simulink library "PB_Library_Master"  (R2020b)
settings: Solver=VariableStepAuto  StartTime=0.0  StopTime=10.0  RelTol=1e-3
undefined symbols (not defined in the file): A_M, B_M, E0_M, f_sw, K_M, Q_M, Q_rr, r_c, r_D, R_M, SOC_Init_M, u_ce0, u_D0
libraries: $bdroot x7, Lib_PF_BusLoadDC_TMATS x3, Lib_Dyn_StateSpace_EMTAT x3, TemperatureBlock x1
(part 2 of 3)

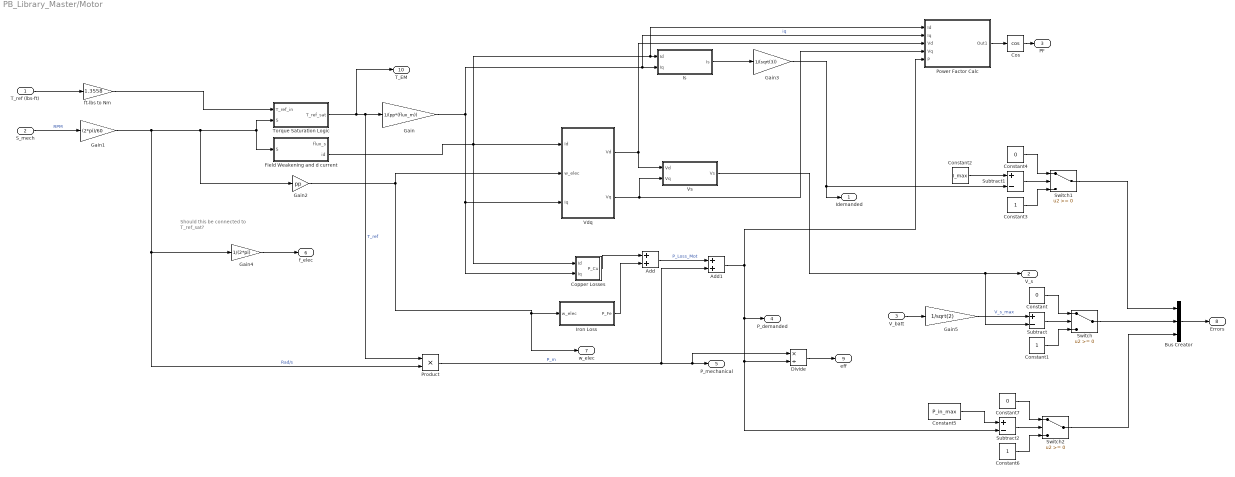
== system PB_Library_Master/Motor ==
  note: Should this be connected
      | to T_ref_sat?
  T_ref (lbs-ft) : Inport
  S_mech : Inport  Port=2
  V_batt : Inport  Port=3
  Add : Sum
  Add1 : Sum
  Bus Creator : BusCreator  Inputs=3
  Constant : Constant  Value=0
  Constant1 : Constant
  Constant2 : Constant  Value=I_max
  Constant3 : Constant
  Constant4 : Constant  Value=0
  Constant5 : Constant  Value=P_in_max
  Constant6 : Constant
  Constant7 : Constant  Value=0
  Copper Losses : Subsystem
  Cos : Trigonometry  Operator=cos
  Divide : Product  Inputs=*/
  "Field Weakening and d current " : Subsystem
  Gain : Gain  Gain=1/(pp*(flux_m))
  Gain1 : Gain  Gain=(2*pi)/60
  Gain2 : Gain  Gain=pp
  Gain3 : Gain  Gain=1/(sqrt(3))
  Gain4 : Gain  Gain=1/(2*pi)
  Gain5 : Gain  Gain=1/sqrt(2)
  Iron Loss : Subsystem
  Is : Subsystem
  "Power Factor Calc " : Subsystem
  Product : Product
  Subtract : Sum  Inputs=+-
  Subtract1 : Sum  Inputs=+-
  Subtract2 : Sum  Inputs=+-
  Switch : Switch
  Switch1 : Switch
  Switch2 : Switch
  Torque Saturation Logic : Subsystem
  Vdq : Subsystem
  Vs : Subsystem
  ft-lbs to Nm : Gain  Gain=1.3558
  Idemanded : Outport  VectorParamsAs1DForOutWhenUnconnected=off
  V_s : Outport  Port=2  VectorParamsAs1DForOutWhenUnconnected=off
  PF : Outport  Port=3  VectorParamsAs1DForOutWhenUnconnected=off
  P_demanded : Outport  Port=4  VectorParamsAs1DForOutWhenUnconnected=off
  P_mechanical : Outport  Port=5  VectorParamsAs1DForOutWhenUnconnected=off
  f_elec : Outport  Port=6  VectorParamsAs1DForOutWhenUnconnected=off
  w_elec : Outport  Port=7  VectorParamsAs1DForOutWhenUnconnected=off
  Errors : Outport  Port=8  VectorParamsAs1DForOutWhenUnconnected=off
  eff : Outport  Port=9  VectorParamsAs1DForOutWhenUnconnected=off
  T_EM : Outport  Port=10  VectorParamsAs1DForOutWhenUnconnected=off
  wires:
  S_mech/1 -> Gain1/1  "RPM"
  T_ref (lbs-ft)/1 -> ft-lbs to Nm/1
  "Field Weakening and d current "/2(id) -> Copper Losses/1(Id), "Power Factor Calc "/1(Id), Is/1(Id), Vdq/1(Id)
  Gain3/1 -> Subtract1/2, Idemanded/1
  Gain2/1 -> Vdq/2(w_elec), w_elec/1, Iron Loss/1(w_elec)
  Torque Saturation Logic/1(T_ref_sat) -> T_EM/1, Product/1, Gain/1  "T_ref"
  Gain/1 -> "Power Factor Calc "/2(Iq), Is/2(Iq), Copper Losses/2(Iq), Vdq/3(Iq)  "iq"
  Gain1/1 -> Gain4/1, Product/2, Gain2/1, "Field Weakening and d current "/1(S), Torque Saturation Logic/2(S)  "Rad/s"
  Copper Losses/1(P_Cu) -> Add/1
  Iron Loss/1(P_Fe) -> Add/2
  Add/1 -> Add1/1  "P_Loss_Mot"
  Product/1 -> Add1/2, Divide/1, P_mechanical/1  "P_m"
  Vdq/1(Vd) -> Vs/1(Vd), "Power Factor Calc "/3(Vd)
  Vdq/2(Vq) -> "Power Factor Calc "/4(Vq), Vs/2(Vq)
  Is/1(Is) -> Gain3/1
  Vs/1(Vs) -> Subtract/2, V_s/1
  "Power Factor Calc "/1(Out1) -> Cos/1
  Add1/1 -> Divide/2, Subtract2/2, P_demanded/1, "Power Factor Calc "/5(P)
  Gain4/1 -> f_elec/1
  V_batt/1 -> Gain5/1
  Gain5/1 -> Subtract/1  "V_s_max"
  Subtract/1 -> Switch/2
  Constant/1 -> Switch/1
  Constant1/1 -> Switch/3
  Switch/1 -> Bus Creator/2
  Constant2/1 -> Subtract1/1
  Switch1/1 -> Bus Creator/1
  Constant3/1 -> Switch1/3
  Constant4/1 -> Switch1/1
  Subtract1/1 -> Switch1/2
  Constant7/1 -> Switch2/1
  Constant5/1 -> Subtract2/1
  Subtract2/1 -> Switch2/2
  Constant6/1 -> Switch2/3
  Divide/1 -> eff/1
  Cos/1 -> PF/1
  Bus Creator/1 -> Errors/1
  Switch2/1 -> Bus Creator/3
  ft-lbs to Nm/1 -> Torque Saturation Logic/1(T_ref_in)

== system PB_Library_Master/Rankine to Celsius ==
  Rankine : Inport
  Add : Sum  Inputs=+-
  Constant : Constant  Value=491.67
  Constant1 : Constant  Value=1.8
  Divide : Product  Inputs=*/
  Celsius : Outport
  wires:
  Divide/1 -> Celsius/1
  Rankine/1 -> Add/1
  Constant/1 -> Add/2
  Add/1 -> Divide/1
  Constant1/1 -> Divide/2

== system PB_Library_Master/Resistor_I ==
  Iout : Inport
  Idemand : Inport  Port=2
  Temp (Rankine) : Inport  Port=3  Unit=degC
  Multiply : Product
  Multiply1 : Product
  Rankine to Celsius : $bdroot/Rankine to Celsius  SystemSampleTime=-1  VariantActivationTime=update diagram  Latency=0  AutoFrameSizeCalculation=off
  Terminator : Terminator
  VDrop : Outport  VectorParamsAs1DForOutWhenUnconnected=off
  Iin : Outport  Port=2  VectorParamsAs1DForOutWhenUnconnected=off
  Heat : Outport  Port=3  VectorParamsAs1DForOutWhenUnconnected=off
  wires:
  Iout/1 -> Multiply/2, Multiply1/2, Iin/1
  Multiply/1 -> VDrop/1, Multiply1/1
  Idemand/1 -> Multiply/1
  Multiply1/1 -> Heat/1
  Temp (Rankine)/1 -> Rankine to Celsius/1
  Rankine to Celsius/1 -> Terminator/1

== system PB_Library_Master/Resistor_V ==
  "VDrop " : Inport
  "Resistance " : Inport  Port=2
  Temp : Inport  Port=3  Unit=degC
  Divide : Product  Inputs=*/
  Multiply1 : Product
  Rankine to Celsius : $bdroot/Rankine to Celsius  SystemSampleTime=-1  VariantActivationTime=update diagram  Latency=0  AutoFrameSizeCalculation=off
  Terminator : Terminator
  Iin : Outport  VectorParamsAs1DForOutWhenUnconnected=off
  Heat : Outport  Port=2  VectorParamsAs1DForOutWhenUnconnected=off
  wires:
  Multiply1/1 -> Heat/1
  "VDrop "/1 -> Multiply1/1, Divide/1
  "Resistance "/1 -> Divide/2
  Divide/1 -> Multiply1/2, Iin/1
  Temp/1 -> Rankine to Celsius/1
  Rankine to Celsius/1 -> Terminator/1

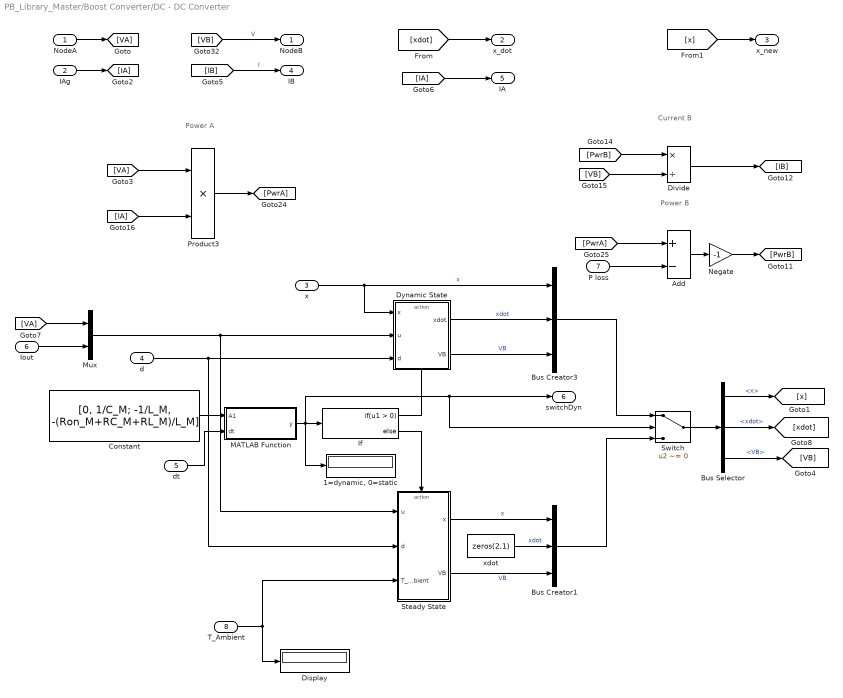
== system PB_Library_Master/Boost Converter/DC - DC Converter ==
  note: Power B
  note: Current B
  note: Power A
  NodeA : Inport
  IAg : Inport  Port=2
  x : Inport  Port=3
  d : Inport  Port=4
  dt : Inport  Port=5
  Iout : Inport  Port=6
  P loss : Inport  Port=7
  "T_Ambient " : Inport  Port=8
  " Dynamic State" : Subsystem  TreatAsAtomicUnit=on
  "1=dynamic, 0=static" : Display
  Add : Sum  Inputs=+-
  Bus Creator1 : BusCreator  Inputs=3
  Bus Creator3 : BusCreator  Inputs=3
  Bus Selector : BusSelector  OutputSignals=x,xdot,VB
  Constant : Constant  Value=[0, 1/C_M; -1/L_M, -(Ron_M+RC_M+RL_M)/L_M]  VectorParams1D=off
  Display : Display
  Divide : Product  Inputs=*/
  If : If
  MATLAB Function : MATLAB Function  TreatAsAtomicUnit=on
  Mux : Mux  Inputs=2
  Negate : Gain  Gain=-1
  Product3 : Product
  Steady State : Subsystem  TreatAsAtomicUnit=on
  Switch : Switch  Criteria=u2 ~= 0
  xdot : Constant  Value=zeros(2,1)  VectorParams1D=off
  NodeB : Outport  VectorParamsAs1DForOutWhenUnconnected=off
  x_dot : Outport  Port=2  VectorParamsAs1DForOutWhenUnconnected=off
  x_new : Outport  Port=3  VectorParamsAs1DForOutWhenUnconnected=off
  IB : Outport  Port=4  VectorParamsAs1DForOutWhenUnconnected=off
  IA : Outport  Port=5  VectorParamsAs1DForOutWhenUnconnected=off
  switchDyn : Outport  Port=6  VectorParamsAs1DForOutWhenUnconnected=off
  wires:
  "T_Ambient "/1 -> Steady State/3("T_Ambient "), Display/1
  Negate/1 -> [PwrB]
  Mux/1 -> " Dynamic State"/2(u), Steady State/1(u)
  Iout/1 -> Mux/2
  [VA] -> Mux/1
  [x] -> x_new/1
  Bus Creator3/1 -> Switch/1
  Bus Selector/1 -> [x]  "<x>"
  Bus Selector/2 -> [xdot]  "<xdot>"
  Bus Selector/3 -> [VB]  "<VB>"
  xdot/1 -> Bus Creator1/2  "xdot"
  Steady State/2(VB) -> Bus Creator1/3  "VB"
  " Dynamic State"/1(xdot) -> Bus Creator3/2  "xdot"
  " Dynamic State"/2(VB) -> Bus Creator3/3  "VB"
  Switch/1 -> Bus Selector/1
  Add/1 -> Negate/1
  P loss/1 -> Add/2
  [PwrA] -> Add/1
  [xdot] -> x_dot/1
  d/1 -> " Dynamic State"/3(d), Steady State/2(d)
  x/1 -> " Dynamic State"/1(x), Bus Creator3/1  "x"
  Steady State/1(x) -> Bus Creator1/1  "x"
  dt/1 -> MATLAB Function/2(dt)
  If/2 -> Steady State/Action
  Constant/1 -> MATLAB Function/1(A1)
  If/1 -> " Dynamic State"/Action
  MATLAB Function/1(y) -> If/1, switchDyn/1, Switch/2, "1=dynamic, 0=static"/1
  [IA] -> IA/1
  [IB] -> IB/1  "I"
  IAg/1 -> [IA]
  [VB] -> Divide/2
  Divide/1 -> [IB]
  [PwrB] -> Divide/1
  [IA] -> Product3/2
  NodeA/1 -> [VA]
  [VB] -> NodeB/1  "V"
  Product3/1 -> [PwrA]
  [VA] -> Product3/1
  Bus Creator1/1 -> Switch/3

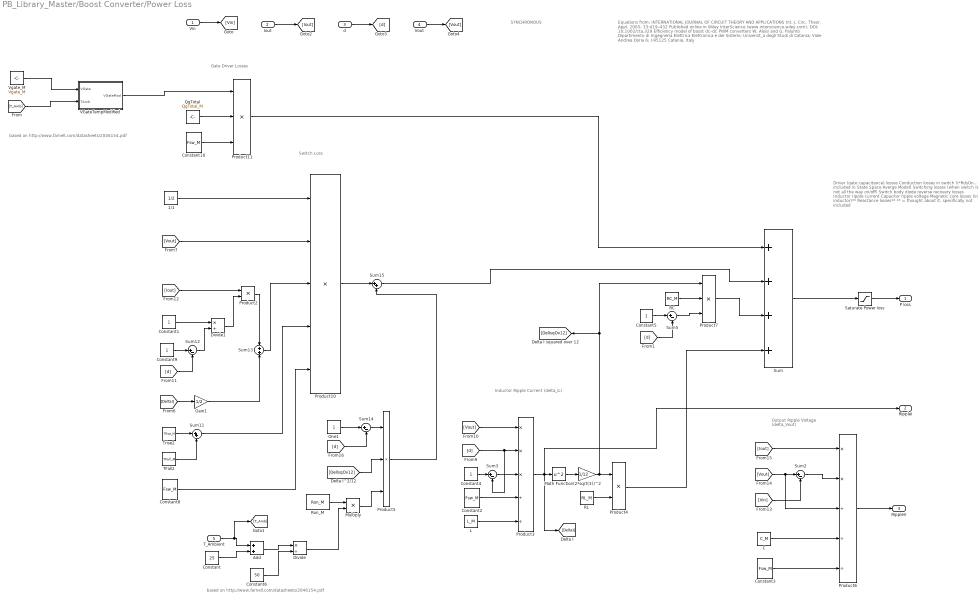
== system PB_Library_Master/Boost Converter/Power Loss  ==
  note: Gate Driver Losses
  note: Output Ripple Voltage
      | (delta_Vout)
  note: Inductor Ripple Current
      | (delta_iL)
  note: Driver (gate capacitance) losses
      | Conduction losses in switch (I*RdsOn... included in State Space Averge Model)
      | Switching losses (when switch is not all the way on/off)
      | Switch body diode reverse recovery losses
      | Inductor ripple current
      | Capacitor ripple voltage
      | Magnetic core losses (in inductor)**
      | Reactance losses**
      | ** = thought about it, specifically not included
  note: SYNCHRONOUS
  note: Switch Loss
  note: Equations from:
      | INTERNATIONAL JOURNAL OF CIRCUIT THEORY AND APPLICATIONS
      | Int. J. Circ. Theor. Appl. 2005; 33:419–432
      | Published online in Wiley InterScience (www.interscience.wiley.com). DOI: 10.1002/cta.329
      | Efficiency model of boost dc–dc PWM converters
      | W. Aloisi and G. Palumb
      | Dipartimento di Ingegneria Elettrica Elettronica e dei Sistemi; Universit_a degli Studi di Catania;
      | Viale Andrea Doria 6; I-95125 Catania, Italy
  note: based on http://www.farnell.com/datasheets/2046154.pdf
  note: based on http://www.farnell.com/datasheets/2046154.pdf
  Vin : Inport
  Iout : Inport  Port=2
  d : Inport  Port=3
  Vout : Inport  Port=4
  "T_Ambient " : Inport  Port=5
  (2*sqrt(3))^2 : Gain  Gain=1/12
  1/1 : Constant  Value=1/2  VectorParams1D=off
  Add : Sum
  C : Constant  Value=C_M  VectorParams1D=off
  Constant : Constant  Value=25
  Constant{1,4..5,9} (4 alike) : Constant
  Constant{2..3,8,10} (4 alike) : Constant  Value=Fsw_M
  Constant6 : Constant  Value=50
  Divide : Product  Inputs=*/
  Divide1 : Product  Inputs=*/
  Gain1 : Gain  Gain=1/2
  L : Constant  Value=L_M  VectorParams1D=off
  Math Function : Math  Operator=square  SignedPower=on  SaturateOnIntegerOverflow=on
  Multiply : Product
  One1 : Constant  VectorParams1D=off
  Product10 : Product  Inputs=5
  Product11 : Product  Inputs=3
  Product2 : Product
  Product3 : Product  Inputs=***//
  Product4 : Product
  Product5 : Product  Inputs=3
  Product6 : Product  Inputs=**///
  Product7 : Product  Inputs=3
  QgTotal : Constant  Value=QgTotal_M  VectorParams1D=off
  RC : Constant  Value=RC_M  VectorParams1D=off
  RL : Constant  Value=RL_M  VectorParams1D=off
  Ron_M : Constant  Value=Ron_M
  Saturate Power loss : Saturate  UpperLimit=inf  LowerLimit=0
  Sum : Sum  Inputs=++++
  Sum11 : Sum  Inputs=|++
  Sum{2..3,5,12,14} (5 alike) : Sum  Inputs=|+-
  Sum13 : Sum
  Sum15 : Sum  Inputs=|++
  TFall2 : Constant  Value=TFall_M  VectorParams1D=off
  Trise2 : Constant  Value=TRise_M  VectorParams1D=off
  VGateTempModified : Subsystem
  "Vgate_M " : Constant  Value=Vgate_M
  " P loss" : Outport  VectorParamsAs1DForOutWhenUnconnected=off
  RippleI : Outport  Port=2  VectorParamsAs1DForOutWhenUnconnected=off
  RippleV : Outport  Port=3  VectorParamsAs1DForOutWhenUnconnected=off
  wires:
  VGateTempModified/1(VGateMod) -> Product11/1
  [T_Amb] -> VGateTempModified/2(TAmb)
  "Vgate_M "/1 -> VGateTempModified/1(VGate)
  Multiply/1 -> Product5/3
  Divide/1 -> Multiply/2
  Add/1 -> Divide/1
  Constant6/1 -> Divide/2
  Constant/1 -> Add/2
  "T_Ambient "/1 -> Add/1, [T_Amb]
  Sum15/1 -> Sum/2
  Product11/1 -> Sum/1
  Product7/1 -> Sum/3
  Product4/1 -> Sum/4
  QgTotal/1 -> Product11/2
  Constant10/1 -> Product11/3
  Product5/1 -> Sum15/2
  Product10/1 -> Sum15/1
  [DelIsqOv12] -> Product5/2
  Sum14/1 -> Product5/1
  Ron_M/1 -> Multiply/1
  One1/1 -> Sum14/1
  [d] -> Sum14/2
  Product6/1 -> RippleV/1
  Constant3/1 -> Product6/5
  C/1 -> Product6/4
  Sum2/1 -> Product6/2
  [Vin] -> Sum2/2
  [Vout] -> Sum2/1, Product6/3
  [Iout] -> Product6/1
  1/1/1 -> Product10/1
  [Vout] -> Product10/2
  Constant8/1 -> Product10/5
  Product2/1 -> Sum13/1
  Sum11/1 -> Product10/4
  Constant1/1 -> Divide1/1
  Trise2/1 -> Sum11/1
  TFall2/1 -> Sum11/2
  Divide1/1 -> Product2/2
  Sum12/1 -> Divide1/2
  Sum13/1 -> Product10/3
  Gain1/1 -> Sum13/2
  Constant9/1 -> Sum12/1
  [d] -> Sum12/2
  [DeltaI] -> Gain1/1
  [Iout] -> Product2/1
  Sum5/1 -> Product7/3
  [d] -> Sum5/2
  Constant5/1 -> Sum5/1
  Sum3/1 -> Product3/3
  Constant4/1 -> Sum3/1
  [Vout] -> Product3/1
  Constant2/1 -> Product3/4
  L/1 -> Product3/5
  Vout/1 -> [Vout]
  [d] -> Product3/2, Sum3/2
  d/1 -> [d]
  Iout/1 -> [Iout]
  Vin/1 -> [Vin]
  Sum/1 -> Saturate Power loss/1
  Saturate Power loss/1 -> " P loss"/1
  RL/1 -> Product4/2
  Product3/1 -> RippleI/1, Math Function/1, [DeltaI]
  (2*sqrt(3))^2/1 -> [DelIsqOv12], Product7/1, Product4/1
  Math Function/1 -> (2*sqrt(3))^2/1
  RC/1 -> Product7/2

== system PB_Library_Master/Boost Converter/TempConv  ==
  Selected Input Units : Inport
  Unit Conversion : UnitConversion
  CelsiusOut : Outport  Unit=°C  VectorParamsAs1DForOutWhenUnconnected=off
  wires:
  Unit Conversion/1 -> CelsiusOut/1  "Celsius"
  Selected Input Units/1 -> Unit Conversion/1

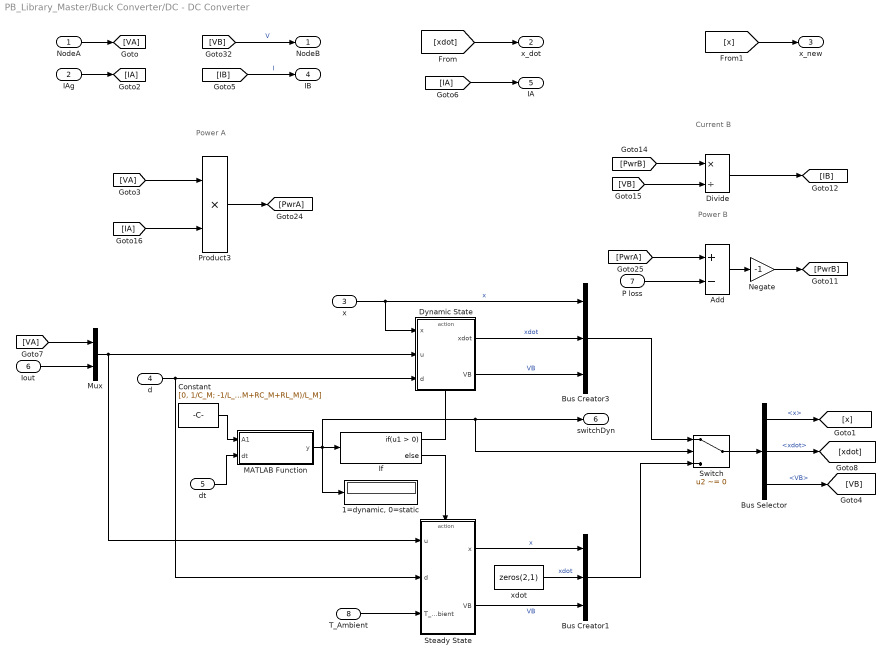
== system PB_Library_Master/Buck Converter/DC - DC Converter ==
  note: Power B
  note: Current B
  note: Power A
  NodeA : Inport
  IAg : Inport  Port=2
  x : Inport  Port=3
  d : Inport  Port=4
  dt : Inport  Port=5
  Iout : Inport  Port=6
  P loss : Inport  Port=7
  "T_Ambient " : Inport  Port=8
  " Dynamic State" : Subsystem  TreatAsAtomicUnit=on
  "1=dynamic, 0=static" : Display
  Add : Sum  Inputs=+-
  Bus Creator1 : BusCreator  Inputs=3
  Bus Creator3 : BusCreator  Inputs=3
  Bus Selector : BusSelector  OutputSignals=x,xdot,VB
  Constant : Constant  Value=[0, 1/C_M; -1/L_M, -(Ron_M+RC_M+RL_M)/L_M]  VectorParams1D=off
  Divide : Product  Inputs=*/
  If : If
  MATLAB Function : MATLAB Function  TreatAsAtomicUnit=on
  Mux : Mux  Inputs=2
  Negate : Gain  Gain=-1
  Product3 : Product
  Steady State : Subsystem  TreatAsAtomicUnit=on
  Switch : Switch  Criteria=u2 ~= 0
  xdot : Constant  Value=zeros(2,1)  VectorParams1D=off
  NodeB : Outport  VectorParamsAs1DForOutWhenUnconnected=off
  x_dot : Outport  Port=2  VectorParamsAs1DForOutWhenUnconnected=off
  x_new : Outport  Port=3  VectorParamsAs1DForOutWhenUnconnected=off
  IB : Outport  Port=4  VectorParamsAs1DForOutWhenUnconnected=off
  IA : Outport  Port=5  VectorParamsAs1DForOutWhenUnconnected=off
  switchDyn : Outport  Port=6  VectorParamsAs1DForOutWhenUnconnected=off
  wires:
  "T_Ambient "/1 -> Steady State/3("T_Ambient ")
  Negate/1 -> [PwrB]
  Mux/1 -> " Dynamic State"/2(u), Steady State/1(u)
  Iout/1 -> Mux/2
  [VA] -> Mux/1
  [x] -> x_new/1
  Bus Creator3/1 -> Switch/1
  Bus Selector/1 -> [x]  "<x>"
  Bus Selector/2 -> [xdot]  "<xdot>"
  Bus Selector/3 -> [VB]  "<VB>"
  xdot/1 -> Bus Creator1/2  "xdot"
  Steady State/2(VB) -> Bus Creator1/3  "VB"
  " Dynamic State"/1(xdot) -> Bus Creator3/2  "xdot"
  " Dynamic State"/2(VB) -> Bus Creator3/3  "VB"
  Switch/1 -> Bus Selector/1
  Add/1 -> Negate/1
  P loss/1 -> Add/2
  [PwrA] -> Add/1
  [xdot] -> x_dot/1
  d/1 -> " Dynamic State"/3(d), Steady State/2(d)
  x/1 -> " Dynamic State"/1(x), Bus Creator3/1  "x"
  Steady State/1(x) -> Bus Creator1/1  "x"
  dt/1 -> MATLAB Function/2(dt)
  If/2 -> Steady State/Action
  Constant/1 -> MATLAB Function/1(A1)
  If/1 -> " Dynamic State"/Action
  MATLAB Function/1(y) -> If/1, switchDyn/1, Switch/2, "1=dynamic, 0=static"/1
  [IA] -> IA/1
  [IB] -> IB/1  "I"
  IAg/1 -> [IA]
  [VB] -> Divide/2
  Divide/1 -> [IB]
  [PwrB] -> Divide/1
  [IA] -> Product3/2
  NodeA/1 -> [VA]
  [VB] -> NodeB/1  "V"
  Product3/1 -> [PwrA]
  [VA] -> Product3/1
  Bus Creator1/1 -> Switch/3

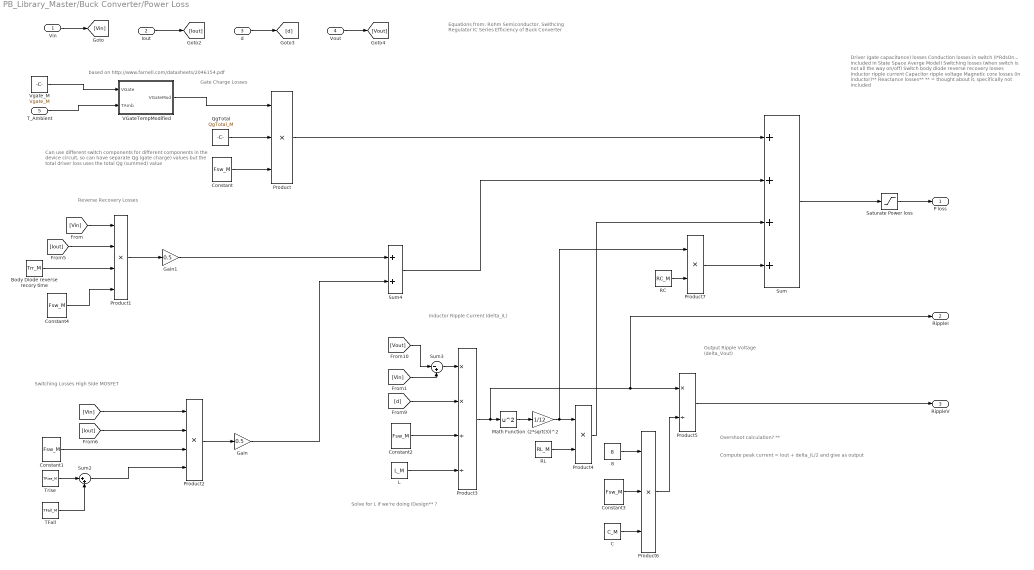
== system PB_Library_Master/Buck Converter/Power Loss  ==
  note: based on http://www.farnell.com/datasheets/2046154.pdf
  note: Overshoot calculation? **
  note: Output Ripple Voltage
      | (delta_Vout)
  note: Inductor Ripple Current
      | (delta_iL)
  note: Reverse Recovery Losses
  note: Switching Losses High Side MOSFET
  note: Driver (gate capacitance) losses
      | Conduction losses in switch (I*RdsOn... included in State Space Averge Model)
      | Switching losses (when switch is not all the way on/off)
      | Switch body diode reverse recovery losses
      | Inductor ripple current
      | Capacitor ripple voltage
      | Magnetic core losses (in inductor)**
      | Reactance losses**
      | ** = thought about it, specifically not included
  note: Can use different switch components for different components in
      | the device circuit, so can have separate Qg (gate charge) values
      | but the total driver loss uses the total Qg (summed) value
  note: Gate Charge Losses
  note: Solve for L if we're doing iDesign** ?
  note: Compute peak current = Iout + delta_IL/2 and give as output
  note: Equations from:
      | Rohm Semiconductor, Swithcing Regulator IC Series
      | Efficiency of Buck Converter
  Vin : Inport
  Iout : Inport  Port=2
  d : Inport  Port=3
  Vout : Inport  Port=4
  "T_Ambient " : Inport  Port=5
  (2*sqrt(3))^2 : Gain  Gain=1/12
  8 : Constant  Value=8  VectorParams1D=off
  Body Diode reverse recory time : Constant  Value=Trr_M  VectorParams1D=off
  C : Constant  Value=C_M  VectorParams1D=off
  Constant{,1..4} (5 alike) : Constant  Value=Fsw_M
  Gain : Gain  Gain=0.5
  Gain1 : Gain  Gain=0.5
  L : Constant  Value=L_M  VectorParams1D=off
  Math Function : Math  Operator=square  SignedPower=on  SaturateOnIntegerOverflow=on
  Product : Product  Inputs=3
  Product1 : Product  Inputs=4
  Product2 : Product  Inputs=4
  Product3 : Product  Inputs=**//
  Product4 : Product
  Product5 : Product  Inputs=*/
  Product6 : Product  Inputs=3
  Product7 : Product
  QgTotal : Constant  Value=QgTotal_M  VectorParams1D=off
  RC : Constant  Value=RC_M  VectorParams1D=off
  RL : Constant  Value=RL_M  VectorParams1D=off
  Saturate Power loss : Saturate  UpperLimit=inf  LowerLimit=0
  Sum : Sum  Inputs=++++
  Sum2 : Sum  Inputs=|++
  Sum3 : Sum  Inputs=|-+
  Sum4 : Sum
  TFall : Constant  Value=TFall_M  VectorParams1D=off
  Trise : Constant  Value=TRise_M  VectorParams1D=off
  VGateTempModified : Subsystem
  Vgate_M : Constant  Value=Vgate_M
  " P loss" : Outport  VectorParamsAs1DForOutWhenUnconnected=off
  RippleI : Outport  Port=2  VectorParamsAs1DForOutWhenUnconnected=off
  RippleV : Outport  Port=3  VectorParamsAs1DForOutWhenUnconnected=off
  wires:
  VGateTempModified/1("VGateMod ") -> Product/1
  "T_Ambient "/1 -> VGateTempModified/2(TAmb)
  Vgate_M/1 -> VGateTempModified/1("VGate ")
  Gain1/1 -> Sum4/1
  Product1/1 -> Gain1/1
  Constant4/1 -> Product1/4
  Body Diode reverse recory time/1 -> Product1/3
  [Iout] -> Product1/2
  [Vin] -> Product1/1
  Gain/1 -> Sum4/2
  Product2/1 -> Gain/1
  Constant3/1 -> Product6/2
  Constant2/1 -> Product3/3
  Constant1/1 -> Product2/3
  Constant/1 -> Product/3
  [Vout] -> Sum3/1
  Vout/1 -> [Vout]
  [d] -> Product3/2
  d/1 -> [d]
  [Iout] -> Product2/2
  Iout/1 -> [Iout]
  [Vin] -> Sum3/2
  [Vin] -> Product2/1
  Vin/1 -> [Vin]
  Sum/1 -> Saturate Power loss/1
  Saturate Power loss/1 -> " P loss"/1
  QgTotal/1 -> Product/2
  Sum4/1 -> Sum/2
  Trise/1 -> Sum2/1
  TFall/1 -> Sum2/2
  Product/1 -> Sum/1
  Sum2/1 -> Product2/4
  Sum3/1 -> Product3/1
  L/1 -> Product3/4
  Product4/1 -> Sum/3
  RL/1 -> Product4/2
  Product3/1 -> Product5/1, RippleI/1, Math Function/1
  (2*sqrt(3))^2/1 -> Product7/1, Product4/1
  Math Function/1 -> (2*sqrt(3))^2/1
  Product6/1 -> Product5/2
  8/1 -> Product6/1
  C/1 -> Product6/3
  Product5/1 -> RippleV/1
  RC/1 -> Product7/2
  Product7/1 -> Sum/4

== system PB_Library_Master/Buck Converter/TempConv  ==
  Selected Input Units : Inport
  Unit Conversion : UnitConversion
  CelsiusOut : Outport  Unit=°C  VectorParamsAs1DForOutWhenUnconnected=off
  wires:
  Unit Conversion/1 -> CelsiusOut/1  "Celsius"
  Selected Input Units/1 -> Unit Conversion/1

== system PB_Library_Master/Electrothermal_Battery_Model/Battery Core (w// Q) ==
  it_base : Inport
  IgIn : Inport  Port=2
  Tavg : Inport  Port=3
  BatteryCore : Subsystem
  Constant1 : Constant  Value=SOC_Init_M
  Vout : Outport  VectorParamsAs1DForOutWhenUnconnected=off
  SOC : Outport  Port=2  VectorParamsAs1DForOutWhenUnconnected=off
  it : Outport  Port=3  VectorParamsAs1DForOutWhenUnconnected=off
  Heat_Generated : Outport  Port=4  VectorParamsAs1DForOutWhenUnconnected=off
  wires:
  IgIn/1 -> BatteryCore/3("Battery Current (A) ")
  Constant1/1 -> BatteryCore/1("SOC Init (%) ")
  Tavg/1 -> BatteryCore/4("Tavg ")
  it_base/1 -> BatteryCore/2("it base (Ah) ")
  BatteryCore/2(it (Ah)) -> it/1
  BatteryCore/1(Battery Voltage (V)) -> Vout/1
  BatteryCore/3(SOC (%)) -> SOC/1
  BatteryCore/4(Heat_Generated) -> Heat_Generated/1

== system PB_Library_Master/Electrothermal_Battery_Model/TempConv  ==
  Selected Input Units : Inport
  Unit Conversion : UnitConversion
  CelsiusOut : Outport  Unit=°C  VectorParamsAs1DForOutWhenUnconnected=off
  wires:
  Unit Conversion/1 -> CelsiusOut/1  "Celsius"
  Selected Input Units/1 -> Unit Conversion/1

== system PB_Library_Master/Electrothermal_Battery_Model/it_Dot = f(i) ==
  i : Inport
  Convert As/s to Ah/s : Gain  Gain=1/3600
  it_Dot : Outport  VectorParamsAs1DForOutWhenUnconnected=off
  wires:
  Convert As/s to Ah/s/1 -> it_Dot/1
  i/1 -> Convert As/s to Ah/s/1

== system PB_Library_Master/Inverter/Diode Conduction Losses ==
  note: You need to read from graphs:
      |
      | -U_ce0
      | -Rc=dU_ce/dI_c (linear)
      | -U_D0
      | -R_D=dU_D/dI_D (linear)
  I_M : Inport
  PF : Inport  Port=2
  m : Inport  Port=3
  T : Inport  Port=4
  1-D Lookup Table r_D : Lookup_n-D  NumberOfTableDimensions=1  BreakpointsForDimension1=T_M  Table=R_D_M  InternalRulePriority=Speed  RndMeth=Simplest  InputSameDT=on
  1-D Lookup Table u_D0 : Lookup_n-D  NumberOfTableDimensions=1  BreakpointsForDimension1=T_M  Table=u_D_M  InternalRulePriority=Speed  RndMeth=Simplest  InputSameDT=on
  Constant : Constant  Value=1/(2*pi)
  Constant1 : Constant  Value=1/8
  Gain : Gain  Commented=on  Gain=u_D0
  Gain1 : Gain  Gain=1/8
  Gain2 : Gain  Commented=on  Gain=r_D
  Gain3 : Gain  Gain=1/(3*pi)
  Product{,1..4} (5 alike) : Product
  Square : Math  Operator=square  SignedPower=on  SaturateOnIntegerOverflow=on
  Sum : Sum  Inputs=+-
  Sum2 : Sum
  Sum3 : Sum  Inputs=-+
  P_CD : Outport  VectorParamsAs1DForOutWhenUnconnected=off
  wires:
  Product/1 -> Sum2/1
  Product2/1 -> Sum2/2
  Sum2/1 -> P_CD/1
  I_M/1 -> Product3/1  "I_M"
  Product3/1 -> Product/2, Square/1
  Constant/1 -> Sum/1
  PF/1 -> Product1/1
  m/1 -> Product1/2
  Gain1/1 -> Sum/2
  Product1/1 -> Gain3/1, Gain1/1
  Sum/1 -> Product/1
  Square/1 -> Product4/1
  Gain3/1 -> Sum3/1
  Product4/1 -> Product2/1
  Constant1/1 -> Sum3/2
  Sum3/1 -> Product2/2
  T/1 -> 1-D Lookup Table u_D0/1, 1-D Lookup Table r_D/1
  1-D Lookup Table u_D0/1 -> Product3/2
  1-D Lookup Table r_D/1 -> Product4/2

== system PB_Library_Master/Inverter/Diode Switching Losses ==
  note: I_Drrpeak=2Qrr/trr
  note: Worst case - voltage across diode is supply voltage
  Input : Inport
  Constant1 : Constant  Value=f_sw
  Gain : Gain  Gain=.25*Q_rr
  Product2 : Product
  P_rec_D : Outport  VectorParamsAs1DForOutWhenUnconnected=off
  wires:
  Product2/1 -> P_rec_D/1
  Constant1/1 -> Product2/2  "I_M"
  Gain/1 -> Product2/1
  Input/1 -> Gain/1  "V_batt"

== system PB_Library_Master/Inverter/IGBT Conduction Losses ==
  note: You need to read from graphs:
      |
      | -U_ce0
      | -Rc=dU_ce/dI_c (linear)
      | -U_D0
      | -R_D=dU_D/dI_D (linear)
  I_M : Inport
  PF : Inport  Port=2
  m : Inport  Port=3
  T : Inport  Port=4
  1-D Lookup Table r_c : Lookup_n-D  NumberOfTableDimensions=1  BreakpointsForDimension1=T_M  Table=R_c_M  InternalRulePriority=Speed  RndMeth=Simplest  InputSameDT=on
  1-D Lookup Table u_ce0 : Lookup_n-D  NumberOfTableDimensions=1  BreakpointsForDimension1=T_M  Table=u_ce0_M  InternalRulePriority=Speed  RndMeth=Simplest  InputSameDT=on
  Constant : Constant  Value=1/(2*pi)
  Constant1 : Constant  Value=1/8
  Gain : Gain  Commented=on  Gain=u_ce0
  Gain1 : Gain  Gain=1/8
  Gain2 : Gain  Commented=on  Gain=r_c
  Gain3 : Gain  Gain=1/(3*pi)
  Product{,1..4} (5 alike) : Product
  Square : Math  Operator=square  SignedPower=on  SaturateOnIntegerOverflow=on
  Sum : Sum
  Sum2 : Sum
  Sum3 : Sum
  P_CT : Outport  VectorParamsAs1DForOutWhenUnconnected=off
  wires:
  Product/1 -> Sum2/1
  Product2/1 -> Sum2/2
  Sum2/1 -> P_CT/1
  I_M/1 -> Product3/1  "I_M"
  Product3/1 -> Product/2, Square/1
  Constant/1 -> Sum/1
  PF/1 -> Product1/1
  m/1 -> Product1/2
  Gain1/1 -> Sum/2
  Product1/1 -> Gain3/1, Gain1/1
  Sum/1 -> Product/1
  Square/1 -> Product4/1
  Gain3/1 -> Sum3/1
  Product4/1 -> Product2/1
  Constant1/1 -> Sum3/2
  Sum3/1 -> Product2/2
  T/1 -> 1-D Lookup Table u_ce0/1, 1-D Lookup Table r_c/1
  1-D Lookup Table u_ce0/1 -> Product3/2
  1-D Lookup Table r_c/1 -> Product4/2

== system PB_Library_Master/Inverter/IGBT Switching Losses ==
  I_ce : Inport
  T : Inport  Port=2
  1-D Lookup Table E0 : Lookup_n-D  NumberOfTableDimensions=1  BreakpointsForDimension1=T_M  Table=E0_M  InternalRulePriority=Speed  RndMeth=Simplest  InputSameDT=on
  1-D Lookup Table E1 : Lookup_n-D  NumberOfTableDimensions=1  BreakpointsForDimension1=T_M  Table=E1_M  InternalRulePriority=Speed  RndMeth=Simplest  InputSameDT=on
  Add : Sum
  Constant : Constant  Value=f_sw_M
  Product : Product
  Product1 : Product
  P_ST : Outport  VectorParamsAs1DForOutWhenUnconnected=off
  wires:
  Constant/1 -> Product/2
  Product/1 -> P_ST/1
  Add/1 -> Product/1
  I_ce/1 -> Product1/1
  1-D Lookup Table E0/1 -> Add/1
  Product1/1 -> Add/2
  T/1 -> 1-D Lookup Table E0/1, 1-D Lookup Table E1/1
  1-D Lookup Table E1/1 -> Product1/2

== system PB_Library_Master/Inverter/I_Ripple ==
  V_batt : Inport
  "V_M " : Inport  Port=2
  Constant : Constant  Value=L_s_M
  Divide : Product  Inputs=*/
  Gain : Gain  Gain=sqrt(2)
  Gain1 : Gain  Gain=2
  Gain2 : Gain  Gain=f_sw_M
  Product : Product
  Product1 : Product
  Subtract : Sum  Inputs=+-
  Out1 : Outport  VectorParamsAs1DForOutWhenUnconnected=off
  wires:
  "V_M "/1 -> Product/2, Gain/1
  Gain/1 -> Subtract/2
  V_batt/1 -> Subtract/1, Product1/1
  Subtract/1 -> Product/1
  Product/1 -> Divide/1
  Constant/1 -> Gain1/1
  Gain1/1 -> Product1/2
  Product1/1 -> Gain2/1
  Gain2/1 -> Divide/2
  Divide/1 -> Out1/1

== system PB_Library_Master/Inverter/P_in_mot ==
  V_s : Inport
  I : Inport  Port=2
  PF : Inport  Port=3
  Gain : Gain  Gain=sqrt(3)
  Product : Product  Inputs=3
  P_in_mot : Outport  VectorParamsAs1DForOutWhenUnconnected=off
  wires:
  I/1 -> Product/2
  PF/1 -> Product/3
  V_s/1 -> Product/1
  Gain/1 -> P_in_mot/1
  Product/1 -> Gain/1

== system PB_Library_Master/Inverter/mVal ==
  V_s : Inport
  V_batt : Inport  Port=2
  Divide : Product  Inputs=*/
  Gain : Gain  Gain=sqrt(2)
  m : Outport  VectorParamsAs1DForOutWhenUnconnected=off
  wires:
  Divide/1 -> m/1
  V_s/1 -> Gain/1
  Gain/1 -> Divide/1
  V_batt/1 -> Divide/2

== system PB_Library_Master/Motor/Copper Losses ==
  Id : Inport
  Iq : Inport  Port=2
  Gain : Gain  Gain=R_s
  Gain1 : Gain  Gain=R_s
  Square : Math  Operator=square  SignedPower=on  SaturateOnIntegerOverflow=on
  Square1 : Math  Operator=square  SignedPower=on  SaturateOnIntegerOverflow=on
  Sum : Sum
  P_Cu : Outport  VectorParamsAs1DForOutWhenUnconnected=off
  wires:
  Iq/1 -> Square1/1
  Id/1 -> Square/1
  Square/1 -> Gain/1
  Square1/1 -> Gain1/1
  Gain1/1 -> Sum/2
  Gain/1 -> Sum/1
  Sum/1 -> P_Cu/1

== system PB_Library_Master/Motor/Field Weakening and d current  ==
  note: Needs: S_n,flux_m,L_s
  S : Inport
  Constant : Constant  Value=flux_m
  Constant1 : Constant  Value=S_nom
  Divide : Product  Inputs=*/
  Gain : Gain  Gain=1/L_s
  Product : Product
  Subtract : Sum  Inputs=+-
  Switch : Switch  Criteria=u2 > Threshold  Threshold=S_nom
  flux_s : Outport  VectorParamsAs1DForOutWhenUnconnected=off
  id : Outport  Port=2  VectorParamsAs1DForOutWhenUnconnected=off
  wires:
  S/1 -> Divide/2, Switch/2
  Product/1 -> Switch/1
  Constant1/1 -> Divide/1
  Divide/1 -> Product/2
  Constant/1 -> Switch/3, Product/1, Subtract/2
  Switch/1 -> Subtract/1, flux_s/1
  Subtract/1 -> Gain/1
  Gain/1 -> id/1

== system PB_Library_Master/Motor/Iron Loss ==
  w_elec : Inport
  Constant : Constant  Value=S_nom*((2*pi)/60)*pp
  Divide : Product  Inputs=*/
  Gain : Gain  Gain=P_Fe_Nom
  P_Fe : Outport  VectorParamsAs1DForOutWhenUnconnected=off
  wires:
  Gain/1 -> P_Fe/1
  w_elec/1 -> Divide/1
  Constant/1 -> Divide/2
  Divide/1 -> Gain/1

== system PB_Library_Master/Motor/Is ==
  Id : Inport
  Iq : Inport  Port=2
  Add : Sum
  Square : Math  Operator=square  SignedPower=on  SaturateOnIntegerOverflow=on
  Square Root : Sqrt  SaturateOnIntegerOverflow=on
  Square1 : Math  Operator=square  SignedPower=on  SaturateOnIntegerOverflow=on
  Is : Outport  VectorParamsAs1DForOutWhenUnconnected=off
  wires:
  Iq/1 -> Square/1
  Id/1 -> Square1/1
  Square1/1 -> Add/1
  Square/1 -> Add/2
  Add/1 -> Square Root/1
  Square Root/1 -> Is/1

== system PB_Library_Master/Motor/Power Factor Calc  ==
  Id : Inport
  Iq : Inport  Port=2
  Vd : Inport  Port=3
  Vq : Inport  Port=4
  P : Inport  Port=5
  Divide : Product  Inputs=*/
  Product : Product
  Product1 : Product
  Subtract : Sum  Inputs=+-
  Trigonometric Function : Trigonometry  Operator=atan
  Out1 : Outport  VectorParamsAs1DForOutWhenUnconnected=off
  wires:
  Vq/1 -> Product/1
  Id/1 -> Product/2
  Vd/1 -> Product1/1
  Iq/1 -> Product1/2
  Product1/1 -> Subtract/2
  Product/1 -> Subtract/1
  Subtract/1 -> Divide/1
  P/1 -> Divide/2
  Divide/1 -> Trigonometric Function/1
  Trigonometric Function/1 -> Out1/1

== system PB_Library_Master/Motor/Torque Saturation Logic ==
  note: Needs: P_m_max, T_ref_max
  T_ref_in : Inport
  S : Inport  Port=2
  Constant1 : Constant  Value=P_out_max
  Divide : Product  Inputs=*/
  Product : Product
  Saturation : Saturate  UpperLimit=T_nom  LowerLimit=0
  Switch : Switch  Criteria=u2 > Threshold  Threshold=P_out_max
  T_ref_sat : Outport  VectorParamsAs1DForOutWhenUnconnected=off
  wires:
  T_ref_in/1 -> Product/1, Saturation/1
  Constant1/1 -> Divide/1
  S/1 -> Product/2, Divide/2
  Saturation/1 -> Switch/3
  Product/1 -> Switch/2
  Divide/1 -> Switch/1
  Switch/1 -> T_ref_sat/1

== system PB_Library_Master/Motor/Vdq ==
  Id : Inport
  w_elec : Inport  Port=2
  Iq : Inport  Port=3
  Gain : Gain  Gain=R_s
  Gain1 : Gain  Gain=R_s
  Gain2 : Gain  Gain=L_s
  Gain3 : Gain  Gain=flux_m
  Product : Product
  Product1 : Product
  Subtract : Sum  Inputs=+-
  Sum : Sum  Inputs=+++
  Vd : Outport  VectorParamsAs1DForOutWhenUnconnected=off
  Vq : Outport  Port=2  VectorParamsAs1DForOutWhenUnconnected=off
  wires:
  Id/1 -> Product1/1, Gain/1
  Iq/1 -> Gain1/1, Product/2
  w_elec/1 -> Gain3/1, Gain2/1
  Gain/1 -> Subtract/1
  Gain2/1 -> Product/1, Product1/2
  Product/1 -> Subtract/2
  Subtract/1 -> Vd/1
  Product1/1 -> Sum/1
  Gain1/1 -> Sum/2
  Gain3/1 -> Sum/3
  Sum/1 -> Vq/1

== system PB_Library_Master/Motor/Vs ==
  Vd : Inport
  Vq : Inport  Port=2
  Add : Sum
  Square : Math  Operator=square  SignedPower=on  SaturateOnIntegerOverflow=on
  Square Root : Sqrt  SaturateOnIntegerOverflow=on
  Square1 : Math  Operator=square  SignedPower=on  SaturateOnIntegerOverflow=on
  Vs : Outport  VectorParamsAs1DForOutWhenUnconnected=off
  wires:
  Vq/1 -> Square/1
  Vd/1 -> Square1/1
  Square1/1 -> Add/1
  Square/1 -> Add/2
  Add/1 -> Square Root/1
  Square Root/1 -> Vs/1

== system PB_Library_Master/Boost Converter/DC - DC Converter/ Dynamic State ==
  note: On Cycle
  note: Off Cycle
  x : Inport
  u : Inport  Port=2
  d : Inport  Port=3
  Action Port : ActionPort
  Constant : Constant
  Product{,1..3} (4 alike) : Product
  "State Space Model A1, B1, C1, D1" : Lib_Dyn_StateSpace_EMTAT/State Space Model  A_M=[0, 0; 0, -(Ron_M+RL_M)/L_M]  B_M=[0, -1/C_M; 1/L_M, 0]  C_M="[1,  0]"  D_M=[0, RC_M]
  "State Space Model A2, B2, C2, D2" : Subsystem  mask(State Space Model){A_M=[0, 1/C_M; -1/L_M, -(Ron_M+RC_M+RL_M)/L_M], B_M=[0, -1/C_M; 1/L_M, RC_M/L_M], C_M=[1,  RC_M], D_M=[0, -RC_M]}
      mask prompts: A_M "A_M - "A" Matrix"; B_M "B_M - "B" Matrix"; C_M "C_M - "C" Matrix"; D_M "D_M - "D" Matrix"
      mask help:
      | This block represents a state space model that can be placed within an interative subsytem (i.e. the Newton-Raphson solver).
      | The states, x, and inputs, u must be fed into the block. The outputs, y, and state derivatives, x_dot are computed
      | via the standard state space equations. Note that the integrator that computes the states by integrating
      | the state derivatives should be placed outside of the iterative subsystem so that multiple integration steps do not
      | occur per each timestep.
      |
      | Initial conditions must be specified in the integrator blocks, and ABCD matrices specified as block mask parameters.
      mask Display:
      | fprintf('x_dot = Ax+Bu\ny = Cx+Du')
      | port_label('input',1,'x')
      | port_label('input',2,'u')
      | port_label('output',1,'x_dot')
      | port_label('output',2,'y')
  Sum : Sum  Inputs=++|
  Sum1 : Sum  Inputs=++|
  Sum2 : Sum  Inputs=+-
  xdot : Outport  VectorParamsAs1DForOutWhenUnconnected=off
  VB : Outport  Port=2  VectorParamsAs1DForOutWhenUnconnected=off
  wires:
  "State Space Model A1, B1, C1, D1"/1 -> Product/1
  d/1 -> [d]
  Sum2/1 -> Product2/2, Product3/2
  Constant/1 -> Sum2/1
  [x] -> "State Space Model A1, B1, C1, D1"/1
  "State Space Model A1, B1, C1, D1"/2 -> Product1/1
  [u] -> "State Space Model A1, B1, C1, D1"/2
  [d] -> Product1/2, Product/2
  [d] -> Sum2/2
  u/1 -> [u]
  [x] -> "State Space Model A2, B2, C2, D2"/1(x)
  [u] -> "State Space Model A2, B2, C2, D2"/2(u)
  Product3/1 -> Sum1/2
  "State Space Model A2, B2, C2, D2"/2(y) -> Product3/1
  "State Space Model A2, B2, C2, D2"/1(x_dot) -> Product2/1
  Product2/1 -> Sum/2
  x/1 -> [x]
  Product1/1 -> Sum1/1
  Product/1 -> Sum/1
  Sum1/1 -> VB/1  "VB"
  Sum/1 -> xdot/1  "xdot"

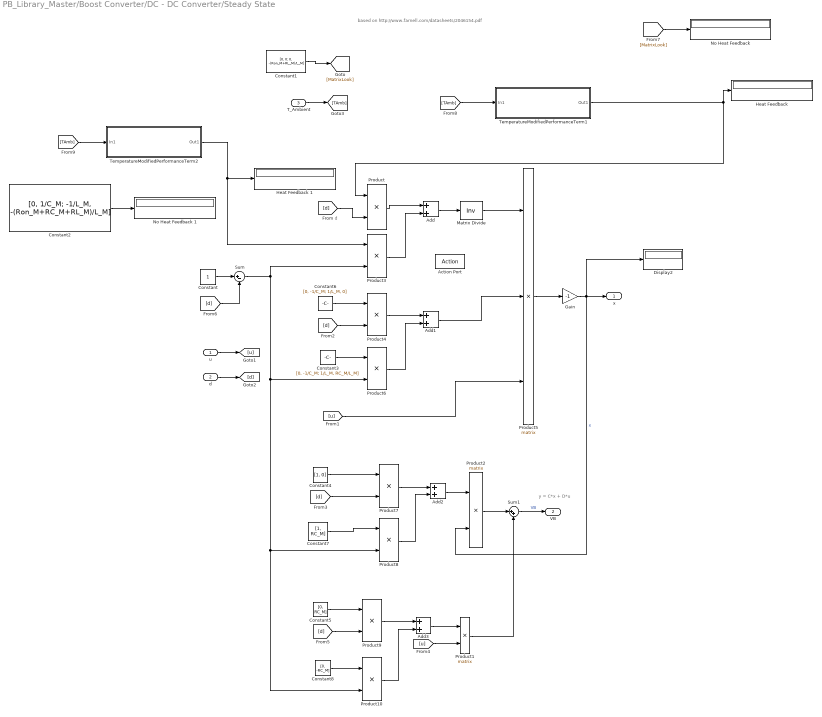
== system PB_Library_Master/Boost Converter/DC - DC Converter/Steady State ==
  note: based on http://www.farnell.com/datasheets/2046154.pdf
  note: d
  note: y = C*x + D*u
  u : Inport
  d : Inport  Port=2
  "T_Ambient " : Inport  Port=3
  Action Port : ActionPort
  Add{,1..3} (4 alike) : Sum
  Constant : Constant
  Constant1 : Constant  Value=[0, 0; 0, -(Ron_M+RL_M)/L_M]  VectorParams1D=off
  Constant2 : Constant  Value=[0, 1/C_M; -1/L_M, -(Ron_M+RC_M+RL_M)/L_M]  VectorParams1D=off
  Constant3 : Constant  Value=[0, -1/C_M; 1/L_M, RC_M/L_M]  VectorParams1D=off
  Constant4 : Constant  Value=[1, 0]  VectorParams1D=off
  Constant5 : Constant  Value=[0, RC_M]  VectorParams1D=off
  Constant6 : Constant  Value=[0, -1/C_M; 1/L_M, 0]  VectorParams1D=off
  Constant7 : Constant  Value=[1, RC_M]  VectorParams1D=off
  Constant8 : Constant  Value=[0, -RC_M]  VectorParams1D=off
  Display2 : Display
  Gain : Gain  Gain=-1
  "Heat Feedback " : Display
  Heat Feedback 1 : Display
  Matrix Divide : Product  Inputs=/  Multiplication=Matrix(*)
  "No Heat Feedback " : Display
  No Heat Feedback 1 : Display
  Product{,3..4,6..10} (8 alike) : Product
  Product1 : Product  Multiplication=Matrix(*)
  Product2 : Product  Multiplication=Matrix(*)
  Product5 : Product  Inputs=3  Multiplication=Matrix(*)
  Sum : Sum  Inputs=|+-
  Sum1 : Sum  Inputs=|++
  "TemperatureModifiedPerformanceTerm1 " : Subsystem
  "TemperatureModifiedPerformanceTerm2 " : Subsystem
  x : Outport  VectorParamsAs1DForOutWhenUnconnected=off
  VB : Outport  Port=2  VectorParamsAs1DForOutWhenUnconnected=off
  wires:
  Constant2/1 -> No Heat Feedback 1/1
  [TAmb] -> "TemperatureModifiedPerformanceTerm2 "/1(In1)
  [TAmb] -> "TemperatureModifiedPerformanceTerm1 "/1(In1)
  "T_Ambient "/1 -> [TAmb]
  "TemperatureModifiedPerformanceTerm2 "/1(Out1) -> Heat Feedback 1/1, Product3/1
  "TemperatureModifiedPerformanceTerm1 "/1(Out1) -> Product/1, "Heat Feedback "/1
  [d] -> Product/2
  [MatrixLook] -> "No Heat Feedback "/1
  Constant8/1 -> Product10/1
  Product6/1 -> Add1/2
  Add/1 -> Matrix Divide/1
  Constant7/1 -> Product8/1
  [d] -> Product7/2
  Add1/1 -> Product5/2
  Product8/1 -> Add2/2
  Product10/1 -> Add3/2
  Constant5/1 -> Product9/1
  [d] -> Sum/2
  Product1/1 -> Sum1/2
  Product5/1 -> Gain/1
  Sum/1 -> Product10/2, Product8/2, Product6/2, Product3/2
  Add3/1 -> Product1/1
  Constant/1 -> Sum/1
  Constant6/1 -> Product4/1
  [u] -> Product5/3
  [d] -> Product4/2
  Gain/1 -> x/1, Display2/1, Product2/2  "x"
  Constant4/1 -> Product7/1
  u/1 -> [u]
  Product2/1 -> Sum1/1
  d/1 -> [d]
  Product7/1 -> Add2/1
  Sum1/1 -> VB/1  "VB"
  Constant1/1 -> [MatrixLook]
  Product4/1 -> Add1/1
  [d] -> Product9/2
  Product/1 -> Add/1
  Constant3/1 -> Product6/1
  Product3/1 -> Add/2
  Matrix Divide/1 -> Product5/1
  Product9/1 -> Add3/1
  Add2/1 -> Product2/1
  [u] -> Product1/2

== system PB_Library_Master/Boost Converter/Power Loss /VGateTempModified ==
  note: normalized to 25°C
  VGate : Inport
  TAmb : Inport  Port=2
  Add1 : Sum
  Constant7 : Constant  Value=25
  Multiply1 : Product
  Subtract : Sum  Inputs=+-
  "V DS temp coefficient " : Constant  Value=.64
  VGateMod : Outport  VectorParamsAs1DForOutWhenUnconnected=off
  wires:
  Add1/1 -> VGateMod/1
  "V DS temp coefficient "/1 -> Multiply1/2
  Subtract/1 -> Multiply1/1
  TAmb/1 -> Subtract/1
  VGate/1 -> Add1/1
  Constant7/1 -> Subtract/2
  Multiply1/1 -> Add1/2

== system PB_Library_Master/Buck Converter/DC - DC Converter/ Dynamic State ==
  x : Inport
  u : Inport  Port=2
  d : Inport  Port=3
  Action Port : ActionPort
  Constant : Constant
  Product{,1..3} (4 alike) : Product
  "State Space Model A1, B1, C1, D1" : Lib_Dyn_StateSpace_EMTAT/State Space Model  A_M=[0, 1/C_M; -1/L_M, -(Ron_M+RC_M+RL_M)/L_M]  B_M=[0, -1/C_M; 1/L_M, RC_M/L_M]  C_M="[1,  RC_M]"  D_M=[0, -RC_M]
  "State Space Model A2, B2, C2, D2" : Lib_Dyn_StateSpace_EMTAT/State Space Model  A_M=[0, 1/C_M; -1/L_M, -(Ron_M+RC_M+RL_M)/L_M]  B_M=[0, -1/C_M; 0, RC_M/L_M]  C_M="[1,  RC_M]"  D_M=[0, -RC_M]
  Sum : Sum  Inputs=++|
  Sum1 : Sum  Inputs=++|
  Sum2 : Sum  Inputs=+-
  xdot : Outport  VectorParamsAs1DForOutWhenUnconnected=off
  VB : Outport  Port=2  VectorParamsAs1DForOutWhenUnconnected=off
  wires:
  "State Space Model A1, B1, C1, D1"/1 -> Product/1
  d/1 -> [d]
  Sum2/1 -> Product2/2, Product3/2
  Constant/1 -> Sum2/1
  [x] -> "State Space Model A1, B1, C1, D1"/1
  "State Space Model A1, B1, C1, D1"/2 -> Product1/1
  [u] -> "State Space Model A1, B1, C1, D1"/2
  [d] -> Product1/2, Product/2
  [d] -> Sum2/2
  u/1 -> [u]
  [x] -> "State Space Model A2, B2, C2, D2"/1
  [u] -> "State Space Model A2, B2, C2, D2"/2
  Product3/1 -> Sum1/2
  "State Space Model A2, B2, C2, D2"/2 -> Product3/1
  "State Space Model A2, B2, C2, D2"/1 -> Product2/1
  Product2/1 -> Sum/2
  x/1 -> [x]
  Product1/1 -> Sum1/1
  Product/1 -> Sum/1
  Sum1/1 -> VB/1  "VB"
  Sum/1 -> xdot/1  "xdot"

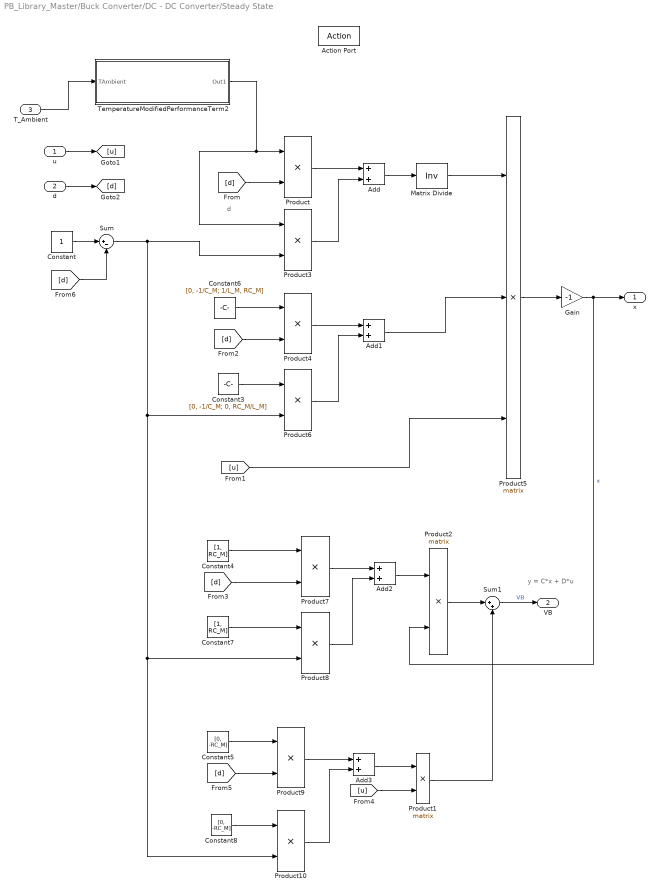
== system PB_Library_Master/Buck Converter/DC - DC Converter/Steady State ==
  note: d
  note: y = C*x + D*u
  u : Inport
  d : Inport  Port=2
  "T_Ambient " : Inport  Port=3
  Action Port : ActionPort
  Add{,1..3} (4 alike) : Sum
  Constant : Constant
  Constant3 : Constant  Value=[0, -1/C_M; 0, RC_M/L_M]  VectorParams1D=off
  Constant4 : Constant  Value=[1, RC_M]  VectorParams1D=off
  Constant5 : Constant  Value=[0, -RC_M]  VectorParams1D=off
  Constant6 : Constant  Value=[0, -1/C_M; 1/L_M, RC_M]  VectorParams1D=off
  Constant7 : Constant  Value=[1, RC_M]  VectorParams1D=off
  Constant8 : Constant  Value=[0, -RC_M]  VectorParams1D=off
  Gain : Gain  Gain=-1
  Matrix Divide : Product  Inputs=/  Multiplication=Matrix(*)
  Product{,3..4,6..10} (8 alike) : Product
  Product1 : Product  Multiplication=Matrix(*)
  Product2 : Product  Multiplication=Matrix(*)
  Product5 : Product  Inputs=3  Multiplication=Matrix(*)
  Sum : Sum  Inputs=|+-
  Sum1 : Sum  Inputs=|++
  "TemperatureModifiedPerformanceTerm2 " : Subsystem
  x : Outport  VectorParamsAs1DForOutWhenUnconnected=off
  VB : Outport  Port=2  VectorParamsAs1DForOutWhenUnconnected=off
  wires:
  "T_Ambient "/1 -> "TemperatureModifiedPerformanceTerm2 "/1(TAmbient)
  "TemperatureModifiedPerformanceTerm2 "/1(Out1) -> Product3/1, Product/1
  Constant8/1 -> Product10/1
  Product6/1 -> Add1/2
  Add/1 -> Matrix Divide/1
  Constant7/1 -> Product8/1
  [d] -> Product7/2
  Add1/1 -> Product5/2
  Product8/1 -> Add2/2
  Product10/1 -> Add3/2
  [d] -> Product/2
  Constant5/1 -> Product9/1
  [d] -> Sum/2
  Product1/1 -> Sum1/2
  Product5/1 -> Gain/1
  Sum/1 -> Product10/2, Product8/2, Product6/2, Product3/2
  Add3/1 -> Product1/1
  Constant/1 -> Sum/1
  Constant6/1 -> Product4/1
  [u] -> Product5/3
  [d] -> Product4/2
  Gain/1 -> x/1, Product2/2  "x"
  Constant4/1 -> Product7/1
  u/1 -> [u]
  Product2/1 -> Sum1/1
  d/1 -> [d]
  Product7/1 -> Add2/1
  Sum1/1 -> VB/1  "VB"
  Product4/1 -> Add1/1
  [d] -> Product9/2
  Product/1 -> Add/1
  Constant3/1 -> Product6/1
  Product3/1 -> Add/2
  Matrix Divide/1 -> Product5/1
  Product9/1 -> Add3/1
  Add2/1 -> Product2/1
  [u] -> Product1/2

== system PB_Library_Master/Buck Converter/Power Loss /VGateTempModified ==
  note: normalized to 25°C
  "VGate " : Inport
  TAmb : Inport  Port=2
  Add1 : Sum
  Constant7 : Constant  Value=25
  Multiply1 : Product
  Subtract : Sum  Inputs=+-
  "V DS temp coefficient " : Constant  Value=.64
  "VGateMod " : Outport  VectorParamsAs1DForOutWhenUnconnected=off
  wires:
  Add1/1 -> "VGateMod "/1
  "V DS temp coefficient "/1 -> Multiply1/2
  Subtract/1 -> Multiply1/1
  TAmb/1 -> Subtract/1
  "VGate "/1 -> Add1/1
  Constant7/1 -> Subtract/2
  Multiply1/1 -> Add1/2

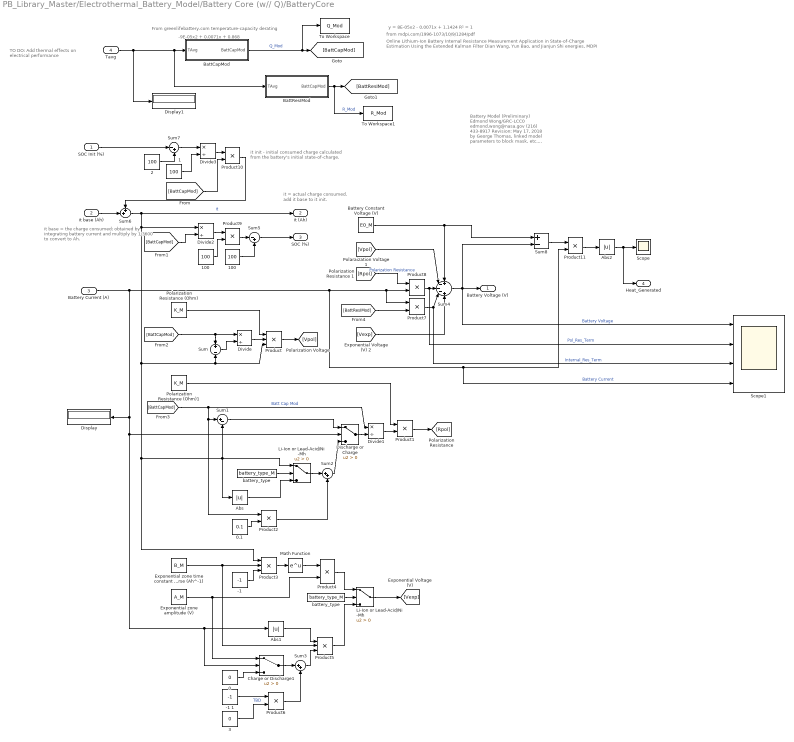
== system PB_Library_Master/Electrothermal_Battery_Model/Battery Core (w// Q)/BatteryCore ==
  note: TO DO: Add thermal effects on electrical performance
  note: it = actual charge consumed.
      | add it base to it init.
  note: it init - initial consumed charge calculated
      | from the battery's initial state-of-charge.
  note: it base = the charge consumed;
      | obtained by integrating battery current
      | and multiply by 1/3600 to convert to Ah.
  note: Battery Model (Preliminary)
      | Edmond Wong/GRC-LCC0
      | edmond.wong@nasa.gov
      | (216) 433-8917
      |
      | Revision: May 17, 2018
      | by George Thomas, linked model
      | parameters to block mask, etc.
      |
      | Revision: April 29, 2019
      | by Mark Bell
      | Heat output, initial temperature feedback
  note: -9E-05x2 + 0.0071x + 0.868
  note: From greenlifebattery.com temperature-capacity derating
  note: y = 8E-05x2 - 0.0071x + 1.1424 R² = 1
  note: from mdpi.com/1996-1073/10/9/1284/pdf
  note: Online Lithium-Ion Battery Internal Resistance Measurement Application in State-of-Charge
      | Estimation Using the Extended Kalman Filter
      |
      | Dian Wang, Yun Bao, and Jianjun Shi
      |
      | energies, MDPI
  "SOC Init (%) " : Inport
  "it base (Ah) " : Inport  Port=2
  "Battery Current (A) " : Inport  Port=3
  "Tavg " : Inport  Port=4
  "-1 " : Constant  Value=-1
  -1 1 : Constant  Value=-1
  0 : Constant  Value=0
  0.1 : Constant  Value=0.1
  1 : Constant  Value=100
  100 : Constant  Value=100
  "100 " : Constant  Value=100
  2 : Constant  Value=100
  3 : Constant  Value=0
  Abs : Abs
  Abs1 : Abs
  Abs2 : Abs
  "BattCapMod " : Subsystem
  "BattResIMod " : Subsystem
  Battery Constant Voltage (V) : Constant  Value=E0_M
  Charge or Discharge1 : Switch  Criteria=u2 > Threshold
  Discharge or Charge : Switch  Criteria=u2 > Threshold
  Display : Display
  Display1 : Display
  Divide{,1..3} (4 alike) : Product  Inputs=*/
  Exponential zone amplitude (V) : Constant  Value=A_M
  Exponential zone time constant inverse (Ah^-1) : Constant  Value=B_M
  Li-Ion or Lead-Acid/Ni-Mh : Switch  Criteria=u2 > Threshold
  "Li-Ion or Lead-Acid/Ni-Mh " : Switch  Criteria=u2 > Threshold
  Math Function : Math  SignedPower=on  SaturateOnIntegerOverflow=on
  Polarization Resistance (Ohm) : Constant  Value=K_M
  Polarization Resistance (Ohm)1 : Constant  Value=K_M
  Product : Product  Inputs=3
  Product{1..2,4,6..11} (9 alike) : Product
  Product3 : Product  Inputs=3
  Product5 : Product  Inputs=3
  Scope : Scope
  Scope1 : Scope  NumInputPorts=4
  Sum : Sum  Inputs=+||-
  Sum1 : Sum  Inputs=|+-
  Sum2 : Sum  Inputs=|++
  Sum3 : Sum  Inputs=|++
  Sum4 : Sum  Inputs=+---+
  Sum5 : Sum  Inputs=|-+
  Sum6 : Sum  Inputs=++|
  Sum7 : Sum  Inputs=|-+
  Sum8 : Sum  Inputs=+-
  To Workspace : ToWorkspace  VariableName=Q_Mod  SampleTime=-1
  To Workspace1 : ToWorkspace  VariableName=R_Mod  SampleTime=-1
  battery_type : Constant  Value=battery_type_M
  "battery_type " : Constant  Value=battery_type_M
  Battery Voltage (V) : Outport  VectorParamsAs1DForOutWhenUnconnected=off
  it (Ah) : Outport  Port=2  VectorParamsAs1DForOutWhenUnconnected=off
  SOC (%) : Outport  Port=3  VectorParamsAs1DForOutWhenUnconnected=off
  Heat_Generated : Outport  Port=4  VectorParamsAs1DForOutWhenUnconnected=off
  wires:
  [BattResIMod] -> Product7/2
  "Tavg "/1 -> Display1/1, "BattCapMod "/1(TAvg), "BattResIMod "/1(TAvg)
  "BattResIMod "/1(BattCapMod) -> To Workspace1/1, [BattResIMod]  "R_Mod"
  [BattCapMod] -> Divide/1, Sum/1
  [BattCapMod] -> Divide2/2
  "BattCapMod "/1(BattCapMod) -> To Workspace/1, [BattCapMod]  "Q_Mod"
  "SOC Init (%) "/1 -> Sum7/1
  Product9/1 -> Sum5/1
  Divide3/1 -> Product10/1
  "100 "/1 -> Sum5/2
  2/1 -> Sum7/2
  Sum7/1 -> Divide3/1
  Product10/1 -> Sum6/1
  "it base (Ah) "/1 -> Sum6/2
  1/1 -> Divide3/2
  Polarization Resistance (Ohm)1/1 -> Product1/1
  Divide/1 -> Product/2
  Product5/1 -> "Li-Ion or Lead-Acid/Ni-Mh "/3
  Product/1 -> [Vpol]
  Sum/1 -> Divide/2
  Product7/1 -> Scope1/3, Sum4/4  "Internal_Res_Term"
  Exponential zone amplitude (V)/1 -> Product4/2, Charge or Discharge1/1
  3/1 -> Product6/2  "TBD"
  Product8/1 -> Scope1/2, Sum4/3  "Pol_Res_Term"
  battery_type/1 -> Li-Ion or Lead-Acid/Ni-Mh/2
  [Vexp] -> Sum4/5
  "battery_type "/1 -> "Li-Ion or Lead-Acid/Ni-Mh "/2
  Product6/1 -> Sum3/2
  Sum6/1 -> Divide2/1, Product/3, Sum/2, Li-Ion or Lead-Acid/Ni-Mh/1, Sum1/2, Abs/1, Product3/1, it (Ah)/1  "it"
  [BattCapMod] -> Divide1/1, Product2/1, Sum1/1  "Batt Cap Mod"
  100/1 -> Product9/2
  "-1 "/1 -> Product3/3
  Charge or Discharge1/1 -> Sum3/1
  Math Function/1 -> Product4/1
  Divide2/1 -> Product9/1
  -1 1/1 -> Product6/1
  [Rpol] -> Product8/1  "Polarization Resistance"
  Sum1/1 -> Discharge or Charge/1
  [Vpol] -> Sum4/2
  Product4/1 -> "Li-Ion or Lead-Acid/Ni-Mh "/1
  Sum5/1 -> SOC (%)/1
  "Li-Ion or Lead-Acid/Ni-Mh "/1 -> [Vexp]
  Polarization Resistance (Ohm)/1 -> Product/1
  Product2/1 -> Sum2/2
  Abs1/1 -> Product5/1
  Discharge or Charge/1 -> Divide1/2
  0/1 -> Charge or Discharge1/3
  Abs/1 -> Li-Ion or Lead-Acid/Ni-Mh/3
  Exponential zone time constant inverse (Ah^-1)/1 -> Product5/2, Product3/2
  Sum2/1 -> Discharge or Charge/3
  Product3/1 -> Math Function/1
  Li-Ion or Lead-Acid/Ni-Mh/1 -> Sum2/1
  Sum3/1 -> Product5/3
  0.1/1 -> Product2/2
  Product1/1 -> [Rpol]
  Divide1/1 -> Product1/2
  Abs2/1 -> Heat_Generated/1, Scope/1
  Sum8/1 -> Product11/1
  Product11/1 -> Abs2/1
  Battery Constant Voltage (V)/1 -> Sum8/1, Sum4/1
  "Battery Current (A) "/1 -> Scope1/4, Product11/2, Product7/1, Product8/2, Discharge or Charge/2, Charge or Discharge1/2, Abs1/1, Display/1  "Battery Current"
  Sum4/1 -> Sum8/2, Battery Voltage (V)/1, Scope1/1  "Battery Voltage"
  [BattCapMod] -> Product10/2

== system PB_Library_Master/Boost Converter/DC - DC Converter/ Dynamic State/State Space Model A2, B2, C2, D2 ==
  note: y = C*x + D*u
  note: x_dot = A*x + B*u
  x : Inport
  u : Inport  Port=2
  Constant : Constant  Value=A_M  VectorParams1D=off
  Constant1 : Constant  Value=B_M  VectorParams1D=off
  Constant2 : Constant  Value=C_M  VectorParams1D=off
  Constant3 : Constant  Value=D_M  VectorParams1D=off
  Display{,1..3} (4 alike) : Display
  Product{1..4} (4 alike) : Product  Multiplication=Matrix(*)
  Sum : Sum  Inputs=|++
  Sum1 : Sum  Inputs=|++
  x_dot : Outport  VectorParamsAs1DForOutWhenUnconnected=off
  y : Outport  Port=2  VectorParamsAs1DForOutWhenUnconnected=off
  wires:
  Sum/1 -> x_dot/1, Display2/1
  x/1 -> [x], Display/1
  Sum1/1 -> y/1, Display3/1
  u/1 -> [u], Display1/1
  Constant/1 -> Product4/1
  [x] -> Product4/2
  [u] -> Product3/2
  Constant1/1 -> Product3/1
  Product4/1 -> Sum/1
  Product3/1 -> Sum/2
  Product2/1 -> Sum1/1
  Constant3/1 -> Product1/1
  [x] -> Product2/2
  Product1/1 -> Sum1/2
  [u] -> Product1/2
  Constant2/1 -> Product2/1

== system PB_Library_Master/Boost Converter/DC - DC Converter/Steady State/TemperatureModifiedPerformanceTerm1  ==
  In1 : Inport
  Add5 : Sum
  Constant11 : Constant  Value=-(L_M)
  Constant13 : Constant  Value=0
  Divide1 : Product  Inputs=*/
  "InductorResistance " : Constant  Value=RL_M
  Matrix Concatenate3 : Concatenate  Mode=Multidimensional array
  Matrix Concatenate4 : Concatenate  Mode=Multidimensional array
  Matrix Concatenate5 : Concatenate  Mode=Multidimensional array  ConcatenateDimension=2
  "TModifiedROn " : Subsystem
  Out1 : Outport  VectorParamsAs1DForOutWhenUnconnected=off
  wires:
  Matrix Concatenate5/1 -> Out1/1
  In1/1 -> "TModifiedROn "/1(In1)
  "InductorResistance "/1 -> Add5/1
  "TModifiedROn "/1(Out1) -> Add5/2
  Constant13/1 -> Matrix Concatenate4/1, Matrix Concatenate4/2, Matrix Concatenate3/1
  Matrix Concatenate4/1 -> Matrix Concatenate5/1
  Divide1/1 -> Matrix Concatenate3/2
  Matrix Concatenate3/1 -> Matrix Concatenate5/2
  Add5/1 -> Divide1/1
  Constant11/1 -> Divide1/2
